simulink library "FG_Controller_Library"  (R2017b)
settings: Solver=VariableStepAuto  StartTime=0.0  StopTime=10.0  RelTol=1e-3
undefined symbols (not defined in the file or in its folder): fcut_velocity_joint, GaitLibrary, isSim, UserParams
libraries: slrtlib x113, simulink x1, func_block_library x1
(part 3 of 3)

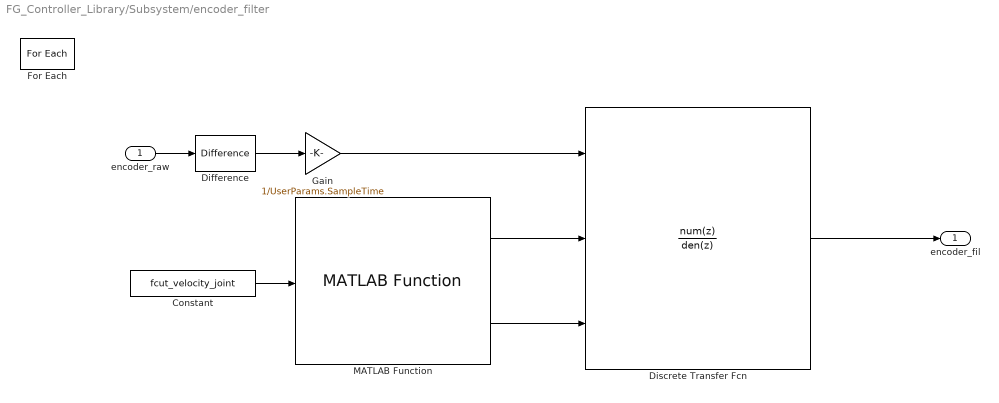
== system FG_Controller_Library/Subsystem/encoder_filter ==
  encoder_raw : Inport  Partition=on  PartitionDimension=1  PartitionWidth=1  PartitionOffset=0
  Constant : Constant  Value=fcut_velocity_joint
  Difference : simulink/Discrete/Difference  ICPrevInput=0.0  OutMin=[]  OutMax=[]  OutDataType=fixdt(1, 16)  OutScaling=2^-10  DoSatur=off
  Discrete Transfer Fcn : DiscreteTransferFcn  NumeratorSource=Input port  DenominatorSource=Input port  SampleTime=UserParams.SampleTime  a0EqualsOne=on
      settings: InputPortMap=u0,p1,p3
  For Each : ForEach  DisableCoverage=on  IndexMode=One-based
  Gain : Gain  Gain=1/UserParams.SampleTime
  MATLAB Function : func_block_library/MATLAB Function
  encoder_fil : Outport  ConcatenationDimension=1
  wires:
  encoder_raw/1 -> Difference/1
  Constant/1 -> MATLAB Function/1
  Difference/1 -> Gain/1
  Gain/1 -> Discrete Transfer Fcn/1
  Discrete Transfer Fcn/1 -> encoder_fil/1
  MATLAB Function/1 -> Discrete Transfer Fcn/2
  MATLAB Function/2 -> Discrete Transfer Fcn/3
